simulink model "ADU_Integration_Y2016_simulation"  (R2016b)
settings: Solver=FixedStepDiscrete  StartTime=240  StopTime=300  FixedStep=0.01  RelTol=1e-3  EnableMultiTasking=on
PostLoadFcn:
  | , if any(exist('dsrtsu_mdlpostloadfcn', 'file') == [2, 3, 6]), try dsrtsu_mdlpostloadfcn('Execute', bdroot); catch fprintf('Error in PostLoadFcn (dsrtsu_mdlpostloadfcn) for model "%s":\n %s\n', bdroot, lasterr); end, end,
InitFcn:
  | load 'data/chi2_dat';
  | load 'data/innerLine_struct';
  | load 'data/middleLine_struct';
  | load 'data/outerLine_struct';
  | load 'data/innerLine';
  | load 'data/middleLine';
  | load 'data/outerLine';
  | load 'data/landmarks_patac_schimmel_ccw';
  | load 'data/patac_navi_array';
  | load 'data/sensor';
  | load 'data/map_struct';
  | addpath map_src
  | Integration_Parameter;
  | load 'TestData_001';
values from neighbouring files (symbols this model uses):
  TestData_001 =     [TestData_001.mat]
undefined symbols (not defined in the file or in its folder): a, chi2_dat, innerLine, landmarks_patac_schimmel_ccw, middleLine, outerLine, patac_navi_array, StartNum
libraries: simulink x36, rtican x1
(part 20 of 20)

== matlab function ADU_Integration_Y2016_simulation/Path_Plan1/LaneChangePathPlanningModule1/PathPrePointCal/PrePointCal ==
  data: xoptres input; x_in input; y_in input; angle_in input; y_out input; angle_out input; Info_Me input; Time input; xposition output; yposition output; Ax output; Ay output; Vx output; Vy output; Theta output; quadcosu2tbl data_store_memory; quadsinu2tbl data_store_memory; PathPlanRes input; PathTrjFinishFlg output
function [xposition,yposition,Ax,Ay,Vx,Vy,Theta,PathTrjFinishFlg] = PosUpdate( xoptres,x_in,y_in,angle_in,y_out,angle_out,Info_Me,Time,PathPlanRes)
persistent PrePointCalEn
if isempty(PrePointCalEn)
    PrePointCalEn = 0;
end
if PrePointCalEn <1e-1
    if PathPlanRes > 1e-1
        PrePointCalEn = 1;
    end
end
xposition = 0;yposition = 0;Ax = 0;Ay = 0;Vx = 0;Vy = 0;Theta = 0;PathTrjFinishFlg = 0;
    DeltaTemp = [0 0];
    k_localmaxTemp = [0 0];
    ArclengthTol = [0 0];
    Arc = 255;
    V_tarPos = 255;
    x_out=xoptres(1);       
    V_me = Info_Me(3);
    if PrePointCalEn > 1e-1
        [ x_qitemp,y_qitemp,theta_qitemp ] = qiConfigCal( x_in,y_in,angle_in,x_out,y_out,angle_out );
        x_qi = x_qitemp;y_qi = y_qitemp;theta_qi = theta_qitemp;
        [DeltaTemp(1),k_localmaxTemp(1),ArclengthTol(1)] = ElementaryPathPlot( x_in,y_in,angle_in,x_qi,y_qi,theta_qi );
        [DeltaTemp(2),k_localmaxTemp(2),ArclengthTol(2)] = ElementaryPathPlot( x_qi,y_qi,theta_qi,x_out,y_out,angle_out );

        V_tar=xoptres(3);
        S_arc = ArclengthTol(1) + ArclengthTol(2);    
        T_long = xoptres(2)*2*S_arc/(V_tar + V_me);
        S_acc = (V_tar + V_me)/2 * T_long;
        S_arc = ArclengthTol(1) + ArclengthTol(2);
        if S_acc < S_arc
            T_lat = T_long + (S_arc - S_acc) / V_tar;
        else
            a = (V_tar - V_me)/T_long;
            V_end = sqrt(V_me^2 + 2*a*S_arc);
            if a == 0
                T_lat = S_arc / V_me;
            else        
                T_lat = (V_end - V_me)/a;
            end
        end

        if Time > T_lat
        else
            if Time <= T_long
                if abs(V_tar - V_me) >1e-5
                    a_me = (V_tar - V_me)/T_long;
                else
                    a_me = 0;
                end
                Arc = V_me * Time + 0.5 * a_me * Time ^2;
                V_tarPos = V_me + Time * a_me;
            else
                Arc = (V_me + V_tar) /2 * T_long + (Time - T_long) * V_tar;            
                V_tarPos = V_tar;
            end
        end

        if Arc <= ArclengthTol(1)
            [xposition,yposition,Theta] = ElementaryPosCal( Arc,DeltaTemp(1),ArclengthTol(1),theta_qitemp,angle_in,x_in,y_in,x_qitemp,y_qitemp );
            if Arc <= ArclengthTol(1)/2
                Kur = Arc * DeltaTemp(1);
            else
                Kur = DeltaTemp(1) * Arc - ArclengthTol(1)/2 * DeltaTemp(1);
            end
        elseif Arc <= (ArclengthTol(1)+ArclengthTol(2))
            Arc = Arc - ArclengthTol(1);
            [xposition,yposition,Theta] = ElementaryPosCal( Arc,DeltaTemp(2),ArclengthTol(2),angle_out,theta_qitemp,x_qitemp,y_qitemp,x_out,y_out );
            if Arc <= ArclengthTol(2)/2
                Kur = Arc * DeltaTemp(2);
            else
                Kur = DeltaTemp(2) * Arc - ArclengthTol(2)/2 * DeltaTemp(2);
            end
            
        else
            V_tarPos = 0;Theta = 0;Kur = 0;Theta = 0;
            PrePointCalEn = 0;
            PathTrjFinishFlg = 1;
        end

        Vx = V_tarPos * cos(Theta);
        Vy = V_tarPos * sin(Theta);
        Arel = V_tarPos^2 * Kur;
        Ax = Arel * cos(Theta);
        Ay = Arel * sin(Theta);
    end
end 
    
function [xposition,yposition,Theta] = ElementaryPosCal( Arc,Delta,Arclength,angle_out,angle_in,x_in,y_in,x_out,y_out )
%UNTITLED Summary of this function goes here
%   Detailed explanation goes here   
    Beta = (angle_out - angle_in)/2;
    theta_rot = angle_in;
    x_outRot = (x_out - x_in)*cos(theta_rot) + (y_out - y_in)*sin(theta_rot);
    y_outRot = (y_out - y_in)*cos(theta_rot) - (x_out - x_in)*sin(theta_rot);    
    if Beta == 0
        SignBeta = 1;
    else
        SignBeta = sign(Beta);
    end
    if Arc < Arclength/2    
        ulimit = Arc * sqrt(abs(Delta)/2);
        Theta = Delta * (Arc)^2/2;
        xpositionTemp = sqrt(2/abs(Delta))*quadcosu2(ulimit);
        ypositionTemp = sqrt(2/abs(Delta))*quadsinu2(ulimit) * SignBeta;
    else
        ulimit = (Arclength - Arc) * sqrt(abs(Delta)/2); 
        %Theta = 2*Beta*SignBeta - Delta * (Arclength - Arc)^2/2; 
        xpositionMirrTemp = sqrt(2/abs(Delta))*quadcosu2(ulimit);
        ypositionMirrTemp = sqrt(2/abs(Delta))*quadsinu2(ulimit) * SignBeta;
        %mirror line Ax+By+C=0
        x_mirr = (x_outRot)/2;
        y_mirr = (y_outRot)/2;
        angle_mirr = pi/2 + atan((y_outRot)/(x_outRot));
        A = tan(angle_mirr);
        B = -1;
        C = y_mirr - A * x_mirr;      
        %two points are symmetrical to the Ax+By+C we just defined
        xpositionTemp = xpositionMirrTemp - 2*A*(A*xpositionMirrTemp+B*ypositionMirrTemp+C)/(A^2+B^2);
        ypositionTemp = ypositionMirrTemp - 2*B*(A*xpositionMirrTemp+B*ypositionMirrTemp+C)/(A^2+B^2);
        Theta = 2*abs(Beta)*SignBeta - Delta * (Arclength - Arc)^2/2;          
    end
    theta_rot = - angle_in;   
    xposition = xpositionTemp*cos(theta_rot) + ypositionTemp*sin(theta_rot);
    yposition = ypositionTemp*cos(theta_rot) - xpositionTemp*sin(theta_rot) ;  
    xposition = xposition + x_in;
    yposition = yposition + y_in;
    Theta = Theta + angle_in;    
end
%#codegen
function [ x_qi,y_qi,theta_qi ] = qiConfigCal( x_in,y_in,angle_in,x_out,y_out,angle_out )
%UNTITLED2 Summary of this function goes here
%   Detailed explanation goes here
    kesi_en = angle_out - angle_in;
    r_en = sqrt((x_in-x_out)^2+(y_in-y_out)^2);
    k_qi_en = 2 * sin(kesi_en/2)/r_en;    
    if k_qi_en == 0
        x_qi = (x_in + x_out)/2;
        y_qi = (y_in + y_out)/2;
        theta_qi = asin((y_out - y_in)/r_en) * 2 + (angle_in + angle_out)/2;        
    else
        r_qi_en = abs(1/k_qi_en);
        angle_qi_CC = 2* asin(r_en*k_qi_en/2);
        alpha_en = atan((y_out-y_in)/(x_out-x_in));
        if (x_out < x_in)
            alpha_en = alpha_en + pi;
        elseif angle_in > pi
            alpha_en = alpha_en + pi*2;
        end
        if alpha_en > 1e-5
            while alpha_en > 2*pi
                alpha_en = alpha_en - 2 * pi;
            end
        else
            while alpha_en < -2*pi
                alpha_en = alpha_en + 2*pi;
            end
        end

        angle_qi = angle_qi_CC/2;
        if k_qi_en == 0
            signK = 1;
        else
            signK = sign(k_qi_en);
        end
        a = r_qi_en * cos(-angle_qi_CC/2+angle_qi)-sqrt(r_qi_en^2-r_en^2/4);
        b = r_qi_en * sin(-angle_qi_CC/2+angle_qi);
        x_qi = a * sin(alpha_en) * signK - b * cos(alpha_en) * signK + (x_in + x_out) / 2;
        y_qi = - a * cos(alpha_en) * signK - b * sin(alpha_en) * signK + (y_in + y_out) / 2 ; 
        theta_qi = - ( angle_in +angle_out )/2 + 2 * alpha_en;
    end
    if theta_qi > 1e-5
        while theta_qi > 2*pi
            theta_qi = theta_qi - 2 * pi;
        end
    else
        while theta_qi < -2*pi
            theta_qi = theta_qi + 2*pi;
        end
    end       
end

function [Delta,k_localmax,Arclength] = ElementaryPathPlot( x_in,y_in,angle_in,x_out,y_out,angle_out )
    %UNTITLED2 Summary of this function goes here
    %   Detailed explanation goes here
    Nlen = 20;
    xposition = zeros(Nlen,1);
    yposition = zeros(Nlen,1);
    Theta = zeros(Nlen,1);
    kur = zeros(Nlen,1);
    %ArcPos = zeros(Nlen,1);
    Beta = (angle_out - angle_in)/2;
    r = sqrt((x_in-x_out)^2+(y_in-y_out)^2);
    %Move
    x_inMove = x_in - x_in;
    y_inMove = y_in - y_in;
    x_outMove = x_out - x_in;
    y_outMove = y_out - y_in;
    %Rotate
    theta_rot = angle_in;
    x_inRot = x_inMove*cos(theta_rot) + y_inMove*sin(theta_rot);
    x_outRot = x_outMove*cos(theta_rot) + y_outMove*sin(theta_rot);
    y_inRot = y_inMove*cos(theta_rot) - x_inMove*sin(theta_rot);
    y_outRot = y_outMove*cos(theta_rot) - x_outMove*sin(theta_rot);    
    SignBeta = sign(Beta);
    Beta = abs(Beta);
    ulimit = sqrt(Beta);
    D_BetaVal = sin(Beta)*quadsinu2(ulimit)+cos(Beta)*quadcosu2(ulimit);
    %Droot = fzero(@(x) sin(x)*quadsinu2(x)+cos(x)*quadcosu2(x), pi);
    Delta = 8*SignBeta*D_BetaVal^2/r^2;
    %longth of the trajectary     
    Arclength = 2*sqrt(2*abs(Beta/Delta*SignBeta));
    k_localmax = Delta * Arclength/2;    
%     ArcPos = 0:(Arclength/Nlen):Arclength;
    %mirror line Ax+By+C=0
%     x_mirr = (x_inRot + x_outRot)/2;
%     y_mirr = (y_inRot + y_outRot)/2;
%     angle_mirr = pi/2 + atan((y_outRot - y_inRot)/(x_outRot - x_inRot));    
%     A = tan(angle_mirr);
%     B = -1;
%     C = y_mirr - A * x_mirr;    
%     for i=1:length(ArcPos)
%         if ArcPos(i)<=Arclength/2
%             ulimit = ArcPos(i) * sqrt(abs(Delta)/2);
%             xposition(i) = sqrt(2/abs(Delta))*quadcosu2(ulimit);
%             yposition(i) = sqrt(2/abs(Delta))*quadsinu2(ulimit) * SignBeta;
%             Theta(i) = Delta * (ArcPos(i))^2/2;
%             kur(i) = ArcPos(i)*Delta;
%             
%         else
%             ulimit = (Arclength - ArcPos(i)) * sqrt(abs(Delta)/2);   
%             xpositionMirrTemp = sqrt(2/abs(Delta))*quadcosu2(ulimit);
%             ypositionMirrTemp = sqrt(2/abs(Delta))*quadsinu2(ulimit) * SignBeta;
%             %two points are symmetrical to the Ax+By+C we just defined
%             xposition(i) = xpositionMirrTemp - 2*A*(A*xpositionMirrTemp+B*ypositionMirrTemp+C)/(A^2+B^2);
%             yposition(i) = ypositionMirrTemp - 2*B*(A*xpositionMirrTemp+B*ypositionMirrTemp+C)/(A^2+B^2);
%             Theta(i) = 2*Beta*SignBeta - Delta * (Arclength - ArcPos(i))^2/2;  
%             kur(i) = (Arclength - ArcPos(i))*Delta;  
%             
%         end
%         %Rotate and move back
%         x_positionMove = xposition(i)*cos(-theta_rot) + yposition(i)*sin(-theta_rot);
%         y_positionMove = yposition(i)*cos(-theta_rot) - xposition(i)*sin(-theta_rot);
% 
%         xposition(i) = x_positionMove + x_in;
%         yposition(i) = y_positionMove + y_in;
%         Theta(i) = Theta(i) + theta_rot;
%     end   
end

function quadcosu2val = quadcosu2( ulimit )
    %UNTITLED4 Summary of this function goes here
    %   Detailed explanation goes here
    % this function is used to calculate the integral of cos(x^2),which is used
    % to calculate x position
    global quadcosu2tbl
    index = fix(ulimit/0.0005) + 1;
    quadcosu2val = quadcosu2tbl(index);
end

function quadsinu2val = quadsinu2( ulimit )
%UNTITLED4 Summary of this function goes here
%   Detailed explanation goes here
% this function is used to calculate the integral of sin(x^2),which is used
% to calculate y position
    global quadsinu2tbl 
    index = fix(ulimit/0.0005) + 1;
    quadsinu2val = quadsinu2tbl(index);
end

== matlab function ADU_Integration_Y2016_simulation/Path_Plan1/LaneChangePathPlanningModule1/PrePointCorConvert/CordConvert ==
  data: xpositionTar input; xpositionPre input; ypositionTar input; ypositionPre input; Ax input; Ay input; Vx input; Vy input; ThetaTar input; xpositionCur input; ypositionCur input; VsPathPlan_h_position output size=[4]; thetaCur input; VsPathPlan_h_Motion output size=[4]; ThetaLo output
function [VsPathPlan_h_position,VsPathPlan_h_Motion,ThetaLo] = ElementaryPosCal( xpositionTar,xpositionPre,ypositionTar,ypositionPre,Ax,Ay,Vx,Vy,ThetaTar,xpositionCur,ypositionCur,thetaCur )
%UNTITLED Summary of this function goes here
%   Detailed explanation goes here

    VsPathPlan_h_position = [0 0 0 0]';
    VsPathPlan_h_Motion = [0 0 0 0]';
    AfterRotX = [0 0 0 0];
    AfterRotY = [0 0 0 0];   
    
    BeforeRotX = [xpositionTar,xpositionPre,Ax,Vx];
    BeforeRotY = [ypositionTar,ypositionPre,Ay,Vy];   
    
    AfterRotX = (BeforeRotX - xpositionCur ) .* cos(thetaCur) + (BeforeRotY - ypositionCur ) .* sin(thetaCur);
    AfterRotY = (BeforeRotY - ypositionCur ) .* cos(thetaCur) - (BeforeRotX - xpositionCur ) .* sin(thetaCur);

    VsPathPlan_h_position(1) = AfterRotX(1);
    VsPathPlan_h_position(2) = AfterRotY(1);
    VsPathPlan_h_position(3) = AfterRotX(2);
    VsPathPlan_h_position(4) = AfterRotY(2);
    
    VsPathPlan_h_Motion(1) = AfterRotX(3);
    VsPathPlan_h_Motion(2) = AfterRotY(3);
    VsPathPlan_h_Motion(3) = AfterRotX(4);
    VsPathPlan_h_Motion(4) = AfterRotY(4);
    ThetaLo = ThetaTar - thetaCur;
    
end

== matlab function ADU_Integration_Y2016_simulation/Path_Plan1/SceneSelectionModule/ObjSelect ==
  data: EgoLane_Index input; Veh_State input; Info_Fd output; Info_Fo output; Info_Ld output; Info_Lo output; Info_Me output; Sur_ObjectId_List input; Object_Info input
function [Info_Fd,Info_Fo,Info_Ld,Info_Lo,Info_Me] = ObjSelect(EgoLane_Index,Veh_State,Sur_ObjectId_List,Object_Info)
    %First Consider 2 lane
    %inter off lane 0
    %inter lane 1 
    %outer lane 2
    %outer off lane 3
    %1st 2nd    
    Info_IndexTemp = [0 0 0 0;0 0 0 0]; 
    ObjNum = 20;
    %Fd Fo Ld Lo
    Info_Tbl = [0 0 0 0 0 0;0 0 0 0 0 0;0 0 0 0 0 0;0 0 0 0 0 0];
    for i = 1:ObjNum
        if Object_Info(i,1)<1e-1
            break;
        else            
            for j = 1:2
                if min(Info_IndexTemp(j,:)) < 1e-1
                    [valtemp, indtemp] = min(abs(Object_Info(i,1) - Sur_ObjectId_List(j,:)));
                    if valtemp < 1e-1
                        Info_IndexTemp(j, indtemp) = i;
                        break;
                    end
                end
            end
        end
    end
    %X Y V L W
    if EgoLane_Index == 1
        DestLane = EgoLane_Index + 1;
    else
        DestLane = EgoLane_Index - 1;
    end
    % DestLane EgoLane DestLane EgoLane 
    IndeMapTbl = [Info_IndexTemp(DestLane,1),Info_IndexTemp(EgoLane_Index,2),Info_IndexTemp(DestLane,2),Info_IndexTemp(EgoLane_Index,1)];
    for i = 1:4    
        if IndeMapTbl(i)>1e-1
            Xtemp = Object_Info(IndeMapTbl(i),2);
            Ytemp = Object_Info(IndeMapTbl(i),4);
            Vxtemp = Object_Info(IndeMapTbl(i),3);
            Vytemp = Object_Info(IndeMapTbl(i),5);
            Ltemp = 2.5;% TBD
            Wtemp =  Object_Info(Info_IndexTemp(EgoLane_Index,1),7);
        else
            if (i == 1)||(i == 2)
                Xtemp = -65535;
                Ytemp = -65535;
                Vxtemp = 65535;
                Vytemp = 65535;
            else
                Xtemp = 65535;
                Ytemp = 65535;
                Vxtemp = 65535;
                Vytemp = 65535;
            end
            Ltemp = 2.5;% TBD
            Wtemp =  0;
        end
        Info_Tbl(i,:) = [Xtemp,Ytemp,sqrt(Vxtemp^2 + Vytemp^2),Ltemp,Wtemp,0];
    end
    Info_Fd = Info_Tbl(1,:);
    Info_Fo = Info_Tbl(2,:);
    Info_Ld = Info_Tbl(3,:);
    Info_Lo = Info_Tbl(4,:);
    Info_Me = [Veh_State(1),Veh_State(2),Veh_State(8),2.5,1.5,0];    
end

== matlab function ADU_Integration_Y2016_simulation/Path_Plan1/SceneSelectionModule/OpSchedule ==
  data: OperationFinishFlg input; Landmark_Info input; Sur_LandmarkIdList input; Navi_LandmarkIdList input; EgoLane_Index input; Curoperation output; OperationLongDislimit output; LandmarkList output; RoadInfo output size=2,4; Info_Fd input; Info_Fo input; Info_Ld input; Info_Lo input; Info_Me input; alivecont output
function [Curoperation,OperationLongDislimit,LandmarkList,RoadInfo,alivecont] = OpSchedule(OperationFinishFlg,Landmark_Info,Sur_LandmarkIdList,Navi_LandmarkIdList,EgoLane_Index,Info_Fd,Info_Fo,Info_Ld,Info_Lo,Info_Me)
    %#codegen
    %OperationFinishFlg 0 NA 1 Success 2 FailtoStart
    persistent NavigationPointFoundFlg NavigationPointTemp OpNextTemp OperationQ aliveconttemp CurNaviPointIndex LandMarkFoundRes; 
    if isempty(aliveconttemp)
        aliveconttemp = 0;
    end
    if isempty(NavigationPointTemp)
        NavigationPointTemp = 0;
    end
    if isempty(OpNextTemp)
        OpNextTemp = 0;
    end
    if isempty(OperationQ)
        OperationQ = [0 0 0 0];
    end
    if isempty(NavigationPointFoundFlg)
        NavigationPointFoundFlg = 0;
    end
    if isempty(CurNaviPointIndex)
        CurNaviPointIndex = 1;
    end
    if isempty(LandMarkFoundRes)
        LandMarkFoundRes = [0 0];
    end
    LCTrigDis = 20;LCTrigVel = 5;OperationLongDislimit = 0;LandMarkNum = 10;NaviPointNum = 20;LandmarkList = [0 0];Landmark_InfoNum = 30;LandMark2Cal_Info = [0 0];Landmark_InfoNum = 8;
    %NeedorNot TransDis
    OpNeedTransition = [1 20;1 20;1 10;0 0;0 0;0 0];RoadInfo = [0 0 0 0;0 0 0 0];
    EgoLaneInfo = [0 0 0 0 0 0];TarLandMarkLaneInfo = [0 0 0 0 0 0];FrontBackFlg = 0;
    %Type 1 Xcross    %Type 2 Tcross    %Type 3 ParkPoint
    %Operation 0 NA    %Operation 1 RT    %Operation 2 LT    %Operation 3 ST    %Operation 4 HT    %Operation 5 LC    %Operation 6 Transition
    NearestLandmark = Sur_LandmarkIdList(1);
    if (OperationFinishFlg == 1)
        if (OperationQ(1) ~= 5)&&(OperationQ(1) ~= 6)&&(OperationQ(1) >1e-1)
            CurNaviPointIndex = CurNaviPointIndex + 1;
            if CurNaviPointIndex > NaviPointNum
                % one circle finished, we need to reinit the path planning
                % module
                CurNaviPointIndex = 1;
            end
        end
            OperationQ(1) = OperationQ(2);OperationQ(2) = OperationQ(3);OperationQ(3) = OperationQ(4);OperationQ(4) = 0;
            if ((OperationQ(2) < 1e-1)&&(OperationQ(3) <1e-1))
                NavigationPointFoundFlg = 0;
            elseif (OperationQ(2) ~= 6)&&(OperationQ(2) ~= 5)
                NavigationPointFoundFlg = 0;
            else
            end
    else  
    end       
    if NavigationPointFoundFlg > 1e-1 
    else
        Navi_NextLandMarkXTemp = Navi_LandmarkIdList(CurNaviPointIndex + 1,1);
        Navi_NextLandMarkYTemp = Navi_LandmarkIdList(CurNaviPointIndex + 1,2);        
        Navi_NextLandMarkRangeTemp = Navi_LandmarkIdList(CurNaviPointIndex + 1,3);   
        Navi_NextLandMarkOPTemp = Navi_LandmarkIdList(CurNaviPointIndex + 1,4);        
        for i = 1: LandMarkNum
            LandmarkTemp = Sur_LandmarkIdList(i);
            if LandmarkTemp < 1e-1
                break;
            else
                LandmarkTypetemp = Landmark_Info(LandmarkTemp,5);  
                MatchRes = Op2LandMarkType(Navi_NextLandMarkOPTemp,LandmarkTypetemp);
                if MatchRes < 1e-1
                else
                    LandmarkXtemp = Landmark_Info(LandmarkTemp,1);
                    LandmarkYtemp = Landmark_Info(LandmarkTemp,2);
                    Dis2Navi = sqrt((LandmarkXtemp - Navi_NextLandMarkXTemp)^2 + (LandmarkYtemp - Navi_NextLandMarkYTemp)^2);
                    if (Dis2Navi - Navi_NextLandMarkRangeTemp) < 0
                        %Need more classify
                        Index = mod(round(LandmarkTypetemp),10);
                        %Judge whether landmark has been passed
                        FrontBackFlg = LandMarkPassByJudgement(LandmarkTemp,Info_Me,Landmark_Info,Landmark_InfoNum);
                        if FrontBackFlg <2
                            LandMarkFoundRes(Index) = LandmarkTemp;
                        end
                    else
                    end
                end
            end
        end
        if (max(LandMarkFoundRes(1)) > 1e-1)&&(max(LandMarkFoundRes(2)) > 1e-1)                         
            NavigationPointFoundFlg = 1;
        else
            LandMarkFoundRes = [0 0];
        end
        if NavigationPointFoundFlg > 1e-1
            LandMarkIdTemp = LandMarkFoundRes(1);
            LandmarkXtemp = (Landmark_Info(LandMarkIdTemp,1)+Landmark_Info(LandMarkIdTemp,3))/2;
            LandmarkYtemp = (Landmark_Info(LandMarkIdTemp,2)+Landmark_Info(LandMarkIdTemp,4))/2;
            OpNextTemp = Navi_NextLandMarkOPTemp;
            if ((OpNeedTransition(OpNextTemp,1)>1e-1))
                Dis2LandMarkTemp = sqrt((LandmarkXtemp - Info_Me(1))^2 + (LandmarkYtemp- Info_Me(2))^2);
                if (Dis2LandMarkTemp <= OpNeedTransition(OpNextTemp,2))
                    if (Dis2LandMarkTemp > (OpNeedTransition(OpNextTemp,2)-1))
                        OperationQ(2) = 6;OperationQ(3) = OpNextTemp;
                    else
                        OperationQ(2) = OpNextTemp;
                    end
                end
            else
                OperationQ(2) = OpNextTemp;
            end
        end
    end
    %update output
    if OperationQ(1) < 1e-1
        LandMarkIdTemp = LandMarkFoundRes(1);
        if LandMarkIdTemp > 1e-1
            LandmarkXtemp = (Landmark_Info(LandMarkIdTemp,1)+Landmark_Info(LandMarkIdTemp,3))/2;
            LandmarkYtemp = (Landmark_Info(LandMarkIdTemp,2)+Landmark_Info(LandMarkIdTemp,4))/2;
            Dis2LandMarkTemp = sqrt((LandmarkXtemp - Info_Me(1))^2 + (LandmarkYtemp- Info_Me(2))^2);
        else
            Dis2LandMarkTemp = 255;
        end
        if (OperationQ(2) > 1e-1) && (Dis2LandMarkTemp > OpNeedTransition(OpNextTemp,2)) || (OperationQ(2) < 1e-1)
            %Judge the Front Car
            %Invalid objstate
            Dis2Obj_Lo = sqrt((Info_Me(1)-Info_Lo(1))^2+(Info_Me(2)-Info_Lo(2))^2);
            %Invalid Front vehicle judgement
            if Info_Lo(1) < 255
                Dis2Lo = sqrt((Info_Lo(1)-Info_Me(1))^2 + (Info_Lo(1)-Info_Me(1))^2);
                if ((Info_Lo(3) < max([(Info_Me(3) - LCTrigVel),0]))&&(Dis2Lo <= LCTrigDis))||(EgoLane_Index > 1)
                    OperationQ(2) = OperationQ(1);OperationQ(3) = OperationQ(2);OperationQ(4) = OperationQ(3);OperationQ(4) = 0;OperationQ(2) = 5;
                    if OpNextTemp > 1e-1
                        OperationLongDislimit = Dis2LandMarkTemp - OpNeedTransition(OpNextTemp,2);
                    end
                else
                end
            else
            end
        end
        OperationQ(1) = OperationQ(2);OperationQ(2) = OperationQ(3);OperationQ(3) = OperationQ(4);OperationQ(4) = 0;                
    end
    Curoperation = OperationQ(1);
    LandmarkList = LandMarkFoundRes;
    %EndLaneExtract
    if Curoperation < 1e-1
    else        
        if abs(Curoperation - 5)<1e-1
            RoadInfo = RoadInfoExtract(Landmark_Info,NearestLandmark,EgoLane_Index,LandmarkList,Info_Me,Curoperation) ;
            OperationLongDislimit = sqrt((RoadInfo(2,1) - Info_Me(1))^2 + (RoadInfo(2,2) - Info_Me(2))^2);      
        else
            RoadInfo = RoadInfoExtract(Landmark_Info,NearestLandmark,EgoLane_Index,LandmarkList,Info_Me,Curoperation) ;
        end
    end
    %limit calculate
    aliveconttemp = aliveconttemp + 1;
    alivecont = aliveconttemp;

end
function FrontBackFlg = LandMarkPassByJudgement(LandmarkTemp,Info_Me,Landmark_Info,Landmark_InfoNum)
    FrontBackFlg = 0;
    LandmarkXtemp = Landmark_Info(LandmarkTemp,1);
    LandmarkYtemp = Landmark_Info(LandmarkTemp,2);
        %Judge whether landmark has been passed
    LandMark2Cal_Info = [LandmarkXtemp,LandmarkYtemp];
    TarLandMarkLaneInfo = TarLandMarkLaneInfoCal(LandmarkTemp,Landmark_InfoNum,Landmark_Info);
    [Distance,DirectionRel2Lane,FrontBackFlg] = LandMarkDisDirCal(TarLandMarkLaneInfo(1),LandMark2Cal_Info,Info_Me); 
end
function MatchRes = Op2LandMarkType(Op,LandmarkType)
%Operation 0 NA    %Operation 1 RT    %Operation 2 LT    %Operation 3 ST    %Operation 4 HT
% XCrossing_Stop (11) % 
% XCrossing_Start (12) % 
% TCrossing_Stop (21)%
% TCrossing_Start (22)%
% ZCrossing (30)%
% Stop_1 (51)%
% Stop_2 (52)%
% LeftTurn_Stop (61)% 
% LeftTurn_Start (62)% 
% RightTurn_Stop (71)% 
% RightTurn_Start (72)% 
% ParkSlotOnRoad_Stop (81)% 
% ParkSlotOnRoad_Start (82)% 
% ParkSlotOffRoad (90)%  
% RoadChange (100)% 
% SpeedLimit (110)%
% GroundArrow (120)%
% TrafficLight (130)%
% UnClassified (180)%
    MatchRes = 0;
    switch (Op)
        case {1,2}
            if LandmarkType < 22
                MatchRes = 1;
            end
        case 3
            if (LandmarkType <= 52)&&(LandmarkType >= 51)
                MatchRes = 1;
            end
        otherwise
    end      
end

function RoadInfo = RoadInfoExtract(Landmark_Info,NearestLandmark,EgoLane_Index,LandmarkList,Info_Me,Curoperation)
    %#codegen
    %OperationFinishFlg 0 NA 1 Success 2 FailtoStart
    % x_out y_out angle_out xlimit
    Landmark_InfoNum = 8;    RoadInfo = [0 0 0 0;0 0 0 0];FailFlg = 0;ForwardStartPoint = 0;BackwardStartPoint = 0;FrontBackFlg = 0;
    EndLandmark = LandmarkList(2);EgoLaneInfo = [0 0 0 0 0 0];TarLandMarkLaneInfo = [0 0 0 0 0 0];
    FrontBackFlg = LandMarkPassByJudgement(NearestLandmark,Info_Me,Landmark_Info,Landmark_InfoNum);
    if FrontBackFlg <2
    else
        NearestLandmark = NearestLandmark + 1;
        if NearestLandmark > Landmark_InfoNum
            NearestLandmark = 1;
        end
    end
    if (abs(Curoperation - 5) > 1e-1)&&(abs(Curoperation - 6) > 1e-1)
        %EndLane Info Calculate
        TarLandMarkLaneInfo = TarLandMarkLaneInfoCal(EndLandmark,Landmark_InfoNum,Landmark_Info);
        %EgoLane Info Calculate
        EgoLaneInfo = EgoLaneInfoCal(NearestLandmark,Landmark_Info,Landmark_InfoNum);        
        RoadInfo(1,:) = [EgoLaneInfo(3),EgoLaneInfo(4),EgoLaneInfo(1),EgoLaneInfo(2)]; 
        RoadInfo(2,:) = [TarLandMarkLaneInfo(5),TarLandMarkLaneInfo(6),TarLandMarkLaneInfo(1),TarLandMarkLaneInfo(2)]; 
    else
        % X_in curlo X_out targetlane Y angle limit
        EgoLaneInfo = EgoLaneInfoCal(NearestLandmark,Landmark_Info,Landmark_InfoNum);
        RoadInfo(1,1) = Info_Me(1);RoadInfo(1,2) = Info_Me(2);RoadInfo(1,3) = Info_Me(6);RoadInfo(1,4) = EgoLaneInfo(2);
        % This is the limit
        RoadInfo(2,:) = [EgoLaneInfo(3),EgoLaneInfo(4),EgoLaneInfo(1),EgoLaneInfo(2)]; 
    end
    %Forward and Backward search for Egolanechange point
    %1 X_in 2 X_out
end
function TarLandMarkLaneInfo = TarLandMarkLaneInfoCal(TarLandmark,Landmark_InfoNum,Landmark_Info)
    IndexStart = TarLandmark;
    TarLandMarkLaneInfo = [0 0 0 0 0 0];
        if TarLandmark < Landmark_InfoNum
            ForwardStartPoint = TarLandmark + 1;                                      
            for i = ForwardStartPoint:Landmark_InfoNum
            %Forward Search for nearest WithChangePoint\
                if (abs(Landmark_Info(i,5) - 100)<1e-1)||(Landmark_Info(i,5) < 22)
                    IndexEnd = i;
                    TarLandMarkLaneInfo = RoadAngleWithCal(IndexStart,IndexEnd,Landmark_Info) 
                    break;
                end
            end
        else
            i = Landmark_InfoNum;            
        end
        if i == Landmark_InfoNum
            ForwardStartPoint = 1;
            for i = ForwardStartPoint:Landmark_InfoNum
            %Forward Search for nearest WithChangePoint\
                if (abs(Landmark_Info(i,5) - 100)<1e-1)||(Landmark_Info(i,5) < 22)
                    IndexEnd = i;
                    TarLandMarkLaneInfo = RoadAngleWithCal(IndexStart,IndexEnd,Landmark_Info) 
                    break;
                end
            end
        end
end
% 1 StartCentPoint(x,y) 2 EndCentPoint(x,y) 3 Angle
function EgoLaneInfo = EgoLaneInfoCal(NearestLandmark,Landmark_Info,Landmark_InfoNum)
    IndexStart = 0;IndexEnd = 0;LaneInfo = [0 0 0 0 0];EgoLaneInfo = [0 0 0 0 0 0];
    if NearestLandmark > 1
            ForwardStartPoint = NearestLandmark;
            BackStartPoint = NearestLandmark - 1;
        else
            ForwardStartPoint = NearestLandmark;
            BackStartPoint = Landmark_InfoNum;
        end
        ForwardEndFlg = 0;
        for i = ForwardStartPoint:Landmark_InfoNum
            if (abs(Landmark_Info(i,5) - 100)<1e-1)||(Landmark_Info(i,5) < 22)     
                IndexEnd = i;
                ForwardEndFlg = 1;
                break;
            end
        end
        if ForwardEndFlg <1e-1
            ForwardStartPoint = 1;
            for i = ForwardStartPoint:Landmark_InfoNum
            %Forward Search for nearest WithChangePoint\
                if (abs(Landmark_Info(i,5) - 100)<1e-1)||(Landmark_Info(i,5) < 22)
                    IndexEnd = i;
                    break;
                end
            end
        end                
        for k = 1:BackStartPoint
            j = BackStartPoint + 1 - k;
            if (abs(Landmark_Info(i,5) - 100)<1e-1)||(Landmark_Info(i,5) < 22)
                IndexStart = j;
                break;
            end
        end
        EgoLaneInfo = RoadAngleWithCal(IndexStart,IndexEnd,Landmark_Info);
end
function RoadInfo = RoadAngleWithCal(IndexStart,IndexEnd,Landmark_Info)
    Distance = 0;LaneAngle=0;RoadInfo = [0 0 0 0 0 0];
    EndCentX = (Landmark_Info(IndexEnd,1) + Landmark_Info(IndexEnd,3))/2;
    EndCentY = (Landmark_Info(IndexEnd,2) + Landmark_Info(IndexEnd,4))/2;
    StartCentX = (Landmark_Info(IndexStart,1) + Landmark_Info(IndexStart,3))/2;
    StartCentY = (Landmark_Info(IndexStart,2) + Landmark_Info(IndexStart,4))/2;   
%     if abs(EndCentX - StartCentX) < 1e-3
%         LaneAngle = pi/2;
%     else
%         LaneAngle = atan((EndCentY - StartCentY)/(EndCentX - StartCentX));
%     end
    Xdis = EndCentX - StartCentX;Ydis = EndCentY - StartCentY;
    [Distance,LaneAngle] = AngleDisCalin2Pi(Xdis,Ydis);
    LaneWith = sqrt((Landmark_Info(IndexEnd,1) - Landmark_Info(IndexEnd,3))^2 + (Landmark_Info(IndexEnd,2) - Landmark_Info(IndexEnd,4))^2);
    RoadInfo = [LaneAngle,LaneWith,EndCentX,EndCentY,StartCentX,StartCentY];
end
%This module had better be judged by the next module
function [OpState] = OpStateJudge(LandMark_InfoSt,LandMarkLane_InfoSt,LandMark_InfoEd,LandMarkLane_InfoEd,Info_Me,Curoperation)
    % 0 Idle(Also indicating the operation is finished) 1 Before Entering 2 During Op     
    persistent CurState
    if isempty(CurState)
        CurState = 0;
    end
    OpState = 0;StopDisTol = 2;HaltDisTol = 2;LCDisTol = 0;TranDisTol = 0;
    %Operation 0 NA    %Operation 1 RT    %Operation 2 LT    %Operation 3 ST    %Operation 4 HT    %Operation 5 LC    %Operation 6 Transition  
    switch  Curoperation
        case {1,2},
            switch CurState
                case {0,1},
                    % Start LandMark Judgement
                    [Distance,DirectionRel2Lane,FrontBackFlg] = LandMarkDisDirCal(LandMarkLane_InfoSt,LandMark_InfoSt,Info_Me);
                    if (FrontBackFlg < 3)&&(FrontBackFlg > 0)
                        CurState = 1;
                    else
                        CurState = 2;
                    end
                case 2,
                    %End LandMark Judgement
                    [Distance,DirectionRel2Lane,FrontBackFlg] = LandMarkDisDirCal(LandMarkLane_InfoEd,LandMark_InfoEd,Info_Me);  
                    if (FrontBackFlg < 3)&&(FrontBackFlg > 0)
                        CurState = 2;
                    else
                        CurState = 0;
                    end
                otherwise,
                    CurState = 0;
            end
        case 3,
            switch CurState
                case {0,1},
                    % Start LandMark Judgement
                    [Distance,DirectionRel2Lane,FrontBackFlg] = LandMarkDisDirCal(LandMarkLane_InfoSt,LandMark_InfoSt,Info_Me);
                    if (FrontBackFlg < 3)&&(FrontBackFlg > 0)
                        CurState = 1;
                    else
                        CurState = 2;
                    end
                case 2,
                    %End LandMark Judgement
                    [Distance,DirectionRel2Lane,FrontBackFlg] = LandMarkDisDirCal(LandMarkLane_InfoEd,LandMark_InfoEd,Info_Me);  
                    %Or quit early? TBD
                    if Distance < StopDisTol
                        CurState = 2;
                    else
                        CurState = 1;
                    end
                otherwise,
                    CurState = 0;
            end                
        case 4,
            switch CurState
                case {0,1},
                    % Start LandMark Judgement
                    [Distance,DirectionRel2Lane,FrontBackFlg] = LandMarkDisDirCal(LandMarkLane_InfoSt,LandMark_InfoSt,Info_Me);
                    if Distance < HaltDisTol
                        CurState = 2;
                    else
                        CurState = 1;
                    end
                otherwise,
                    CurState = 0;
            end 
        case 5,
            % This had better to be judged by lower module,cause accucy
            % need to be very high
            
        case 6,
            % This is the same with LC
            
        otherwise
    end
 
end
function [Distance,DirectionRel2Lane,FrontBackFlg] = LandMarkDisDirCal(LandMarkLane_Angle,LandMark2Cal_Info,Info_Me)    
    %1\Calculate angle 2\check direction to lane angle
    % LandMark_Info XcentPos YcentPos
    % Vechicle XcentPos YcentPos
    %Calculate angle
    Xdis = LandMark2Cal_Info(1) - Info_Me(1);
    Ydis = LandMark2Cal_Info(2) - Info_Me(2);
    Distance = 0;DirectionRel2Lane = 0;FrontBackFlg = 0;theta = 0;    
    [Distance,theta] = AngleDisCalin2Pi(Xdis,Ydis);    
    DirectionRel2Lane = theta - LandMarkLane_Angle;    
    %pi/2 3*pi/2 on the point 0-pi/2 and 3*pi/2-2*pi Front
    if (DirectionRel2Lane < pi/2)||(DirectionRel2Lane > 3*pi/2)
        FrontBackFlg = 1;
    elseif (DirectionRel2Lane > pi/2)&&(DirectionRel2Lane < 3*pi/2)
        FrontBackFlg = 3;
    else
        % Forward 1 Backward 3 Onthe Point 2 Invalid 0
        FrontBackFlg = 2;
    end
end
function [Distance,theta] = AngleDisCalin2Pi(Xdis,Ydis)
    theta = 0;
    Distance = sqrt(Xdis^2 + Ydis^2);
    if abs(Xdis) < 1e-5
        if Ydis < 0
            theta = 3*pi/2;
        else
            theta = pi/2;
        end
    else
        theta = atan(Ydis/Xdis);
        if abs(theta)<1e-5
            if Xdis < 0
                theta = pi;
            else
                theta = 0;
            end
        else
            if Xdis < 0
                theta = theta + pi;
            else
                theta = theta + 2*pi;
            end                
        end
    end
end

== matlab function ADU_Integration_Y2016_simulation/map2pathplanning ==
  data: local_landmarks_id_front input; local_landmarks_id_rear input; vehicle_state input; object_list_update input; global_landmarks input; object_of_interest_id input; maneuvers input; ego_lane input; odo_state_v input; Sur_LandmarkIdList_front output; Sur_LandmarkIdList_rear output; Veh_State output; Object_Info output; Sur_ObjectId_List output; Landmark_Info output; Navi_LandmarkIdList output; EgoLane_Index output
function [Sur_LandmarkIdList_front,...
          Sur_LandmarkIdList_rear,...
          Veh_State,...
          Object_Info,...
          Sur_ObjectId_List,...
          Landmark_Info,...
          Navi_LandmarkIdList,...
          EgoLane_Index]  = ...
    map2pp(local_landmarks_id_front,...
            local_landmarks_id_rear,...
            vehicle_state,...
            object_list_update, ...
            global_landmarks,...
            object_of_interest_id, ...
            maneuvers, ...
            ego_lane, ...
            odo_state_v)
        
%         Sur_LandmarkIdList_front = local_landmarks_id_front;
%           Sur_LandmarkIdList_front = local_landmarks_id_rear;
%         Object_Info = object_list_update;
%         Landmark_Info = global_landmarks;
%            
%         Veh_State = zeros(1,8);
%         Veh_State(1:5) = vehicle_state';
%         Veh_State(8) = odo_state_v;
%         Navi_LandmarkIdList = maneuvers;
% 
%         Sur_ObjectId_List = zeros(3,10);
%         Sur_ObjectId_List(1,1) = object_of_interest_id;
%         
%         EgoLane_Index = ego_lane;
%     %#codegen
    OperationFinishFlg = 1;
    Landmark_Info = zeros(30,5);
%     Landmark_Info(1,:) = [0,0,0,-4,12];Landmark_Info(8,:) = [0,0,-4,0,11];
%     Landmark_Info(2,:) = [100,0,100,-4,11];Landmark_Info(3,:) = [100,0,104,0,12];
%     Landmark_Info(4,:) = [100,100,104,100,11];Landmark_Info(5,:) = [100,100,100,104,12];
%     Landmark_Info(6,:) = [0,100,0,104,11];Landmark_Info(7,:) = [0,100,-4,100,12];
%     for i = 1:8 
%         plot(Landmark_Info(i,1),Landmark_Info(i,2),'*',Landmark_Info(i,3),Landmark_Info(i,4),'*');
%         hold on        
%     end
    Landmark_Info(1,:) = [0,0,0,-4,12];Landmark_Info(8,:) = [-20,20,-24,20,11];
    Landmark_Info(2,:) = [100,0,100,-4,11];Landmark_Info(3,:) = [120,20,124,20,12];
    Landmark_Info(4,:) = [120,120,124,120,11];Landmark_Info(5,:) = [100,140,100,144,12];
    Landmark_Info(6,:) = [0,140,0,144,11];Landmark_Info(7,:) = [-20,120,-24,120,12];
    Navi_LandmarkIdList = [0,20,40,2;100,20,40,2;100,120,40,2;0,120,40,2];
    EgoLane_Index = 1;
    Veh_State = [99.5,-2,0,0,0,0,0,0]';
    Sur_ObjectId_List = zeros(3,10);
    Sur_ObjectId_List(1,:) = [1,2,0,0,0,0,0,0,0,0];
    Object_Info = zeros(127,26);
    Object_Info(1,:) = [1,122,0,50,0,1,2.5,0,0,0,0,0,0,0,0,0,1,30,10,0,0,1,2.5,0,0,0;];    
    Object_Info(2,:) = [2,122,0,-50,0,1,2.5,0,0,0,0,0,0,0,0,0,1,30,10,0,0,1,2.5,0,0,0;]; 
    Object_Info(3,:) = [3,30,10,0,0,1,2.5,0,0,0,0,0,0,0,0,0,1,30,10,0,0,1,2.5,0,0,0;];    
    Object_Info(4,:) = [4,30,10,0,0,1,2.5,0,0,0,0,0,0,0,0,0,1,30,10,0,0,1,2.5,0,0,0;]; 
    Sur_LandmarkIdList_front = [2,3,4,5,6,7,8,1,0]';
    Sur_LandmarkIdList_rear = [2,3,4,5,6,7,8,1,0]';
end
